simulink model "model_bez_funkcji"  (R2019b)
settings: Solver=FixedStepDiscrete  StartTime=0.0  StopTime=0.001  FixedStep=10e-9  RelTol=1e-3
settings Model: Creator=bwieczorek  LastModifiedBy=bwieczorek

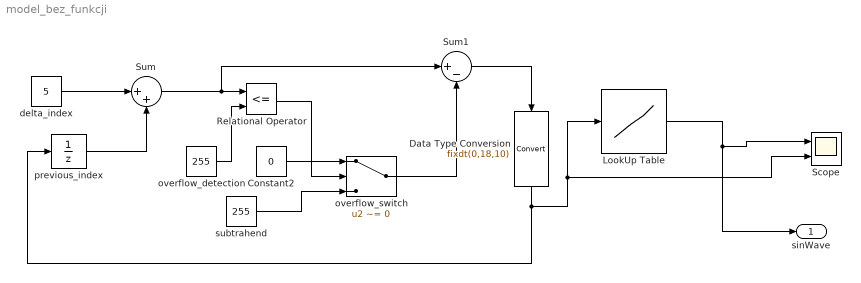
== system model_bez_funkcji ==
  Constant2 : Constant  Value=0  OutDataTypeStr=fixdt(0,18,10)  SampleTime=1e-6
  Data Type Conversion : DataTypeConversion  OutDataTypeStr=fixdt(0,18,10)
  LookUp Table : Lookup_n-D  NumberOfTableDimensions=1  BreakpointsSpecification=Even spacing  BreakpointsForDimension1=[linspace(0, 255, 256)]  BreakpointsForDimension1FirstPoint=0  BreakpointsForDimension1DataTypeStr=fixdt(0,18, 10)  IndexSearchMethod=Linear search  BeginIndexSearchUsingPreviousIndexResult=on  Table=sin([0:0.024639:2*3.141592])  TableDataTypeStr=fixdt(1,18,17)  ExtrapMethod=Clip  RemoveProtectionInput=on  UseLastTableValue=on  InternalRulePriority=Speed  OutDataTypeStr=fixdt(1,18,17)  RndMeth=Simplest  SupportTunableTableSize=on  MaximumIndicesForEachDimension=[255]  InputSameDT=on
  Relational Operator : RelationalOperator  Operator=<=  OutDataTypeStr=boolean  RndMeth=Nearest
  Scope : Scope  NumInputPorts=2
  Sum : Sum  Inputs=|++
  Sum1 : Sum  Inputs=|+-
  delta_index : Constant  Value=5  OutDataTypeStr=fixdt(0,18,10)  SampleTime=1e-6
  overflow_detection : Constant  Value=255  OutDataTypeStr=fixdt(0,18,10)  SampleTime=1e-6  LockScale=on
  overflow_switch : Switch  Criteria=u2 ~= 0
  previous_index : UnitDelay  SampleTime=-1  HasFrameUpgradeWarning=on
  subtrahend : Constant  Value=255  OutDataTypeStr=fixdt(0,18,10)  SampleTime=1e-6
  "sinWave " : Outport  VectorParamsAs1DForOutWhenUnconnected=off
  wires:
  delta_index/1 -> Sum/1
  previous_index/1 -> Sum/2
  Sum/1 -> Sum1/1, Relational Operator/1
  overflow_detection/1 -> Relational Operator/2
  Relational Operator/1 -> overflow_switch/2
  overflow_switch/1 -> Sum1/2
  Constant2/1 -> overflow_switch/1
  subtrahend/1 -> overflow_switch/3
  LookUp Table/1 -> "sinWave "/1, Scope/1
  Sum1/1 -> Data Type Conversion/1
  Data Type Conversion/1 -> previous_index/1, LookUp Table/1, Scope/2
